simulink library "INT_CrCUI"  (R2016b)
settings: Solver=VariableStepAuto  StartTime=0.0  StopTime=10.0  RelTol=1e-3
settings Model: Creator=guanxiaoxing  LastModifiedBy=guanxiaoxing

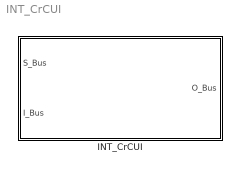
== system INT_CrCUI ==
  INT_CrCUI : Subsystem

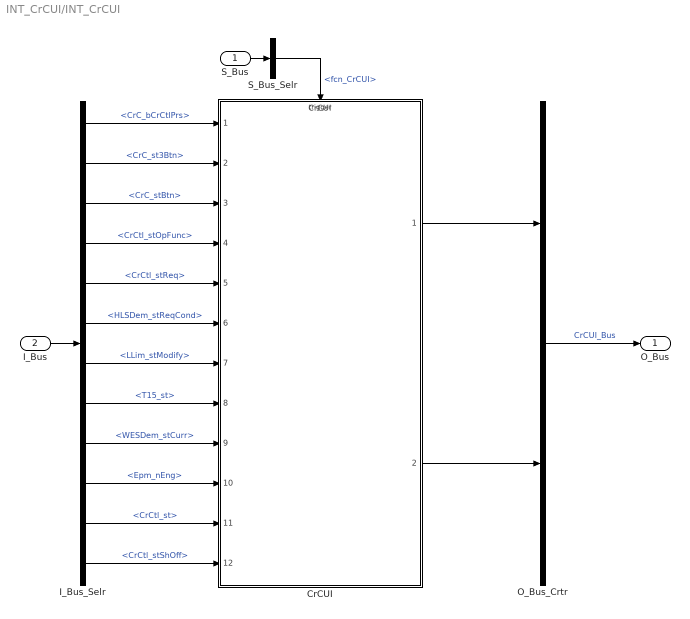
== system INT_CrCUI/INT_CrCUI ==
  S_Bus : Inport
  I_Bus : Inport  Port=2
  CrCUI : ModelReference  ModelNameDialog=CrCUI  SimulationMode=Normal  ModelReferenceVersion=1.60  TriggerPortName=function  TriggerPortTriggerType=function-call  TriggerPortStatesWhenEnabling=held
  I_Bus_Selr : BusSelector  OutputSignals=CrC_bCrCtlPrs,CrC_st3Btn,CrC_stBtn,CrCtl_stOpFunc,CrCtl_stReq,HLSDem_stReqCond,LLim_stModify,T15_st,WESDem_stCurr,Epm_nEng,CrCtl_st,CrCtl_stShOff
  O_Bus_Crtr : BusCreator  Inputs=2
  S_Bus_Selr : BusSelector  OutputSignals=fcn_CrCUI
  O_Bus : Outport
  wires:
  S_Bus_Selr/1 -> CrCUI/Trigger  "<fcn_CrCUI>"
  S_Bus/1 -> S_Bus_Selr/1
  I_Bus/1 -> I_Bus_Selr/1
  I_Bus_Selr/1 -> CrCUI/1  "<CrC_bCrCtlPrs>"
  I_Bus_Selr/2 -> CrCUI/2  "<CrC_st3Btn>"
  I_Bus_Selr/3 -> CrCUI/3  "<CrC_stBtn>"
  I_Bus_Selr/4 -> CrCUI/4  "<CrCtl_stOpFunc>"
  I_Bus_Selr/5 -> CrCUI/5  "<CrCtl_stReq>"
  I_Bus_Selr/6 -> CrCUI/6  "<HLSDem_stReqCond>"
  I_Bus_Selr/7 -> CrCUI/7  "<LLim_stModify>"
  I_Bus_Selr/8 -> CrCUI/8  "<T15_st>"
  I_Bus_Selr/9 -> CrCUI/9  "<WESDem_stCurr>"
  I_Bus_Selr/10 -> CrCUI/10  "<Epm_nEng>"
  I_Bus_Selr/11 -> CrCUI/11  "<CrCtl_st>"
  I_Bus_Selr/12 -> CrCUI/12  "<CrCtl_stShOff>"
  O_Bus_Crtr/1 -> O_Bus/1  "CrCUI_Bus"
  CrCUI/1 -> O_Bus_Crtr/1
  CrCUI/2 -> O_Bus_Crtr/2
